simulink model "HW2_2"  (R2018a)
settings: Solver=VariableStepAuto  StartTime=0.0  StopTime=10.0  RelTol=1e-3
values from neighbouring files (symbols this model uses):
  B = .13    (= 0.13)    [HW2script.m]
  J = .01    (= 0.01)    [HW2script.m]
  K = 52    [HW2script.m]
settings Model: Creator=User  LastModifiedBy=User

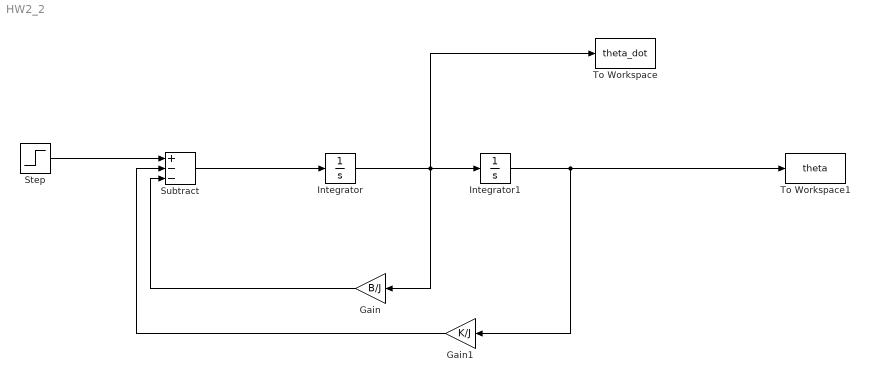
== system HW2_2 ==
  Gain : Gain  Gain=B/J
  Gain1 : Gain  Gain=K/J
  Integrator : Integrator
  Integrator1 : Integrator
  Step : Step  SampleTime=0
  Subtract : Sum  Inputs=+--
  To Workspace : ToWorkspace  VariableName=theta_dot  SaveFormat=Timeseries  SampleTime=-1
  To Workspace1 : ToWorkspace  VariableName=theta  SaveFormat=Timeseries  SampleTime=-1
  wires:
  Gain/1 -> Subtract/3
  Gain1/1 -> Subtract/2
  Integrator/1 -> To Workspace/1, Gain/1, Integrator1/1
  Subtract/1 -> Integrator/1
  Integrator1/1 -> To Workspace1/1, Gain1/1
  Step/1 -> Subtract/1
